simulink model "noise_removal"  (R2013a)
settings: Solver=VariableStepDiscrete  StartTime=0.0  StopTime=0.010  RelTol=1e-3
undefined symbols (not defined in the file or in its folder): xlipgetpartsetting
libraries: xbsIndex_r4 x6, simulink x1
settings Model: Creator=diego  LastModifiedBy=diego

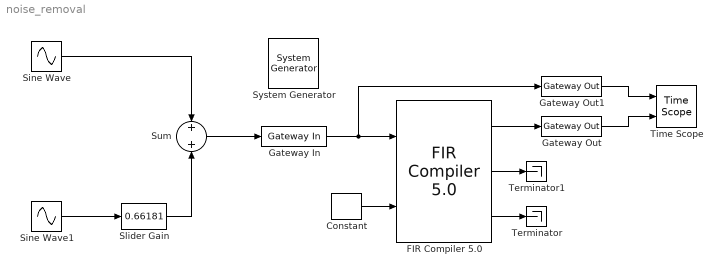
== system noise_removal ==
  " System Generator" : xbsIndex_r4/ System Generator  Tag=genX  xilinxfamily=spartan6  part=xc6slx45t  speed=-3  package=fgg484  synthesis_tool=XST  clock_wrapper=Clock Enables  directory=./netlist  proj_type=Project Navigator  Synth_file=XST Defaults  Impl_file=ISE Defaults  testbench=off  simulink_period=2.0833e-05  sysclk_period=15  dcm_input_clock_period=10  incr_netlist=off  trim_vbits=Everywhere in SubSystem  dbl_ovrd=According to Block Masks  core_generation=According to Block Masks  run_coregen=off  deprecated_control=off  eval_field=0  block_type=sysgen
  Constant : xbsIndex_r4/Constant  const=1  gui_display_data_type=Boolean  arith_type=Boolean  n_bits=16  bin_pt=14  preci_type=Single  exp_width=8  frac_width=24  explicit_period=off  period=1  equ=P=C  opselect=C  inp2=PCIN>>17  opr=+  inp1=P  carry=CIN  dbl_ovrd=off  block_type=constant
  "FIR Compiler 5.0 " : xbsIndex_r4/FIR Compiler 5.0   coefficientvector=[0.0016,0.0013,-0.0005,-0.0037,-0.0055,-0.0018,0.0084,0.0175,0.0133,-0.0103,-0.0406,-0.0482,-0.0053,0.0900,0.2034,0.2804,0.2804,0.2034,0.0900,-0.0053,-0.0482,-0.0406,-0.0103,0.0133,0.0175,0.0084,-0.0018,-0.0055,-0.0037,-0.0005,0.0013,0.0016]  coefficient_sets=1  filter_type=Single_Rate  rate_change_type=Integer  interpolation_rate=1  decimation_rate=1  zero_pack_factor=1  number_channels=1  ratespecification=Sample_Period  sampleperiod=1  hardwareoversamplingrate=1  filter_architecture=Distributed_Arithmetic  coefficient_reload=off  coefficient_structure=Inferred  coefficient_sign=Signed  quantization=Quantize_Only  coefficient_width=16  bestprecision=on  coefficient_fractional_bits=16  number_paths=1  output_rounding_mode=Full_Precision  output_width=37  allow_rounding_approximation=off  optimization_goal=Area  has_sclr=off  has_data_valid=off  has_nd=on  has_ce=off  usechan_in_adv=off  chan_in_adv=0  data_buffer_type=Not_Applicable  coefficient_buffer_type=Not_Applicable  input_buffer_type=Not_Applicable  output_buffer_type=Not_Applicable  preference_for_other_storage=Not_Applicable  multi_column_support=Disabled  columnconfig='1'  inter_column_pipe_length=4  passband_min=0.0  passband_max=0.5  stopband_min=0.5  stopband_max=1.0  filter_selection=1  gui_behaviour=Sysgen  registered_output=true  data_sign=Signed  data_width=16  data_fractional_bits=0  wrapper_available=true  ip_wrap_arbitrary_binary_point=true  ip_name=FIR Compiler  ip_version=5.0  dsptool_ready=true  ipcore_usecache=true  ipcore_useipmodelcache=true  ipcore_xco_need_fpga_part=true  port_translation_map={ 'ce' => 'en', 'sclr' => 'rst' }  run_core_at_system_period=true  ipcore_fpga_part=xlipgetpartsetting(gcb, {'virtex4', 'xc4vsx35', '-10', 'ff668'})  structural_sim=false  block_type=fir_compiler_v5_0
  Gateway In : xbsIndex_r4/Gateway In  gui_display_data_type=Fixed-point  arith_type="Signed  (2's comp)"  n_bits=16  bin_pt=14  preci_type=Single  exp_width=8  frac_width=24  quantization="Round  (unbiased: +/- Inf)"  overflow=Saturate  period=2.0833e-05  dbl_ovrd=off  timing_constraint=None  locs_specified=off  LOCs={}  UseAsADC=off  ADCChannel='1'  inherit_from_input=off  hdl_port=on  block_type=gatewayin
  Gateway Out : xbsIndex_r4/Gateway Out  inherit_from_input=on  hdl_port=on  timing_constraint=None  locs_specified=off  LOCs={}  UseAsDAC=off  DACChannel='1'  block_type=gatewayout
  Gateway Out1 : xbsIndex_r4/Gateway Out  inherit_from_input=off  hdl_port=on  timing_constraint=None  locs_specified=off  LOCs={}  UseAsDAC=off  DACChannel='1'  block_type=gatewayout
  Sine Wave : Sin  Frequency=1e3*2*pi  SampleTime=1/48e3
  Sine Wave1 : Sin  Amplitude=0.5  Frequency=15e3*2*pi  SampleTime=1/48e3
  Slider Gain : simulink/Math Operations/Slider Gain  low=0.24771  gain=0.66181  high=1
  Sum : Sum  Inputs=+|+
  Terminator : Terminator
  Terminator1 : Terminator
  Time Scope : TimeScope  NumInputPorts=2  DefaultConfigurationName=spbscopes.TimeScopeBlockCfg
      settings: CopyFcn=scopeextensions.ScopeBlock.callback(gcbh, 'onBlockCopy', gcbh);  DeleteFcn=scopeextensions.ScopeBlock.callback(gcbh, 'onBlockDelete');  PreSaveFcn=scopeextensions.ScopeBlock.callback(gcbh, 'onModelSave');  NameChangeFcn=scopeextensions.ScopeBlock.callback(gcbh, 'onBlockRename');  CloseFcn=scopeextensions.ScopeBlock.callback(gcbh, 'onBlockClose');  PreDeleteFcn=scopeextensions.ScopeBlock.callback(gcbh, 'onBlockPreDelete');
  wires:
  Sine Wave1/1 -> Slider Gain/1
  Gateway In/1 -> Gateway Out1/1, "FIR Compiler 5.0 "/1
  Constant/1 -> "FIR Compiler 5.0 "/2
  "FIR Compiler 5.0 "/3 -> Terminator/1
  "FIR Compiler 5.0 "/2 -> Terminator1/1
  Sum/1 -> Gateway In/1
  Sine Wave/1 -> Sum/1
  Slider Gain/1 -> Sum/2
  "FIR Compiler 5.0 "/1 -> Gateway Out/1
  Gateway Out/1 -> Time Scope/2
  Gateway Out1/1 -> Time Scope/1
